simulink model "Problem4"  (R2020a)
settings: Solver=VariableStepAuto  StartTime=0.0  StopTime=10.0  RelTol=1e-3
libraries: simulink x1
settings Model: Creator=sreeram  LastModifiedBy=sreeram

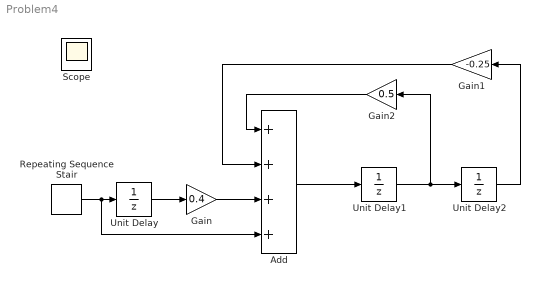
== system Problem4 ==
  Add : Sum  Inputs=++++
  Gain : Gain  Gain=0.4
  Gain1 : Gain  Gain=-0.25
  Gain2 : Gain  Gain=0.5
  Repeating Sequence Stair : simulink/Sources/Repeating Sequence Stair  OutValues=[3 1 4 2 1].'  tsamp=-1  OutMin=[]  OutMax=[]  OutDataTypeStr=double  OutputDataTypeScalingMode=double  OutDataType=fixdt(0,8)  ConRadixGroup=Best Precision: Vector-wise  OutScaling=2^-12
  Unit Delay : UnitDelay  SampleTime=-1  HasFrameUpgradeWarning=on
  Unit Delay1 : UnitDelay  SampleTime=-1  HasFrameUpgradeWarning=on
  Unit Delay2 : UnitDelay  SampleTime=-1  HasFrameUpgradeWarning=on
  Scope : Scope
  wires:
  Repeating Sequence Stair/1 -> Add/4, Unit Delay/1
  Unit Delay/1 -> Gain/1
  Gain/1 -> Add/3
  Add/1 -> Unit Delay1/1
  Unit Delay1/1 -> Gain2/1, Unit Delay2/1
  Unit Delay2/1 -> Gain1/1
  Gain2/1 -> Add/1
  Gain1/1 -> Add/2
